simulink model "ss_ulin"  (Simulink 2.20)
settings: Solver=ode45  StartTime=0.0  StopTime=10.0  RelTol=1e-3  AbsTol=1e-6
values from neighbouring files (symbols this model uses):
  K = acker(Phi, Gamma, pz)    [tilstandmodel_lang_pind.m]
  k1 = 14.69268    [tilstandmodel_lang_pind.m]
  k2 = 1.43688    [tilstandmodel_lang_pind.m]
  k3 = 6.41894    [tilstandmodel_lang_pind.m]
  Keff = 1.3146    [tilstandmodel_lang_pind.m]
  kr1 = Phi_r(2,1)-Lr*Phi_r(1,1)    [tilstandmodel_lang_pind.m]
  kr2 = Phi_r(2,2)-Lr*Phi_r(1,2)    [tilstandmodel_lang_pind.m]
  kr3 = Gamma_r(2)-Lr*Gamma_r(1)    [tilstandmodel_lang_pind.m]
  Lr = (Phi_r(2,2) -pze)/Phi_r(1,2)    [tilstandmodel_lang_pind.m]
  N1 = 14/40    (= 0.35)    [tilstandmodel_lang_pind.m]
  N2 = 12/40    (= 0.3)    [tilstandmodel_lang_pind.m]
libraries: simulink x2
settings Model: ConsistencyChecking=off  RTWPlaceOutputsASAP=off

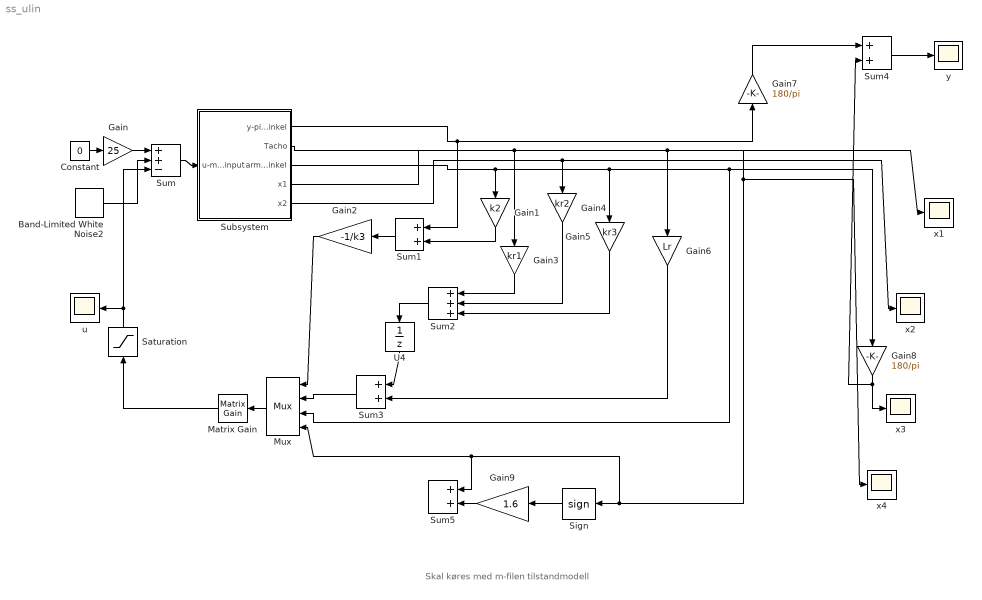
== system ss_ulin ==
  note: Skal køres med m-filen tilstandmodell
  Band-Limited White Noise2 : simulink/Sources/Band-Limited White Noise  Cov=[0.2]  Ts=0.025  seed=[23341]
  Constant : Constant  Value=0
  Gain : Gain  Gain=25
  Gain1 : Gain  Orientation=down  Gain=k2
  Gain2 : Gain  Orientation=left  Gain=-1/k3
  Gain3 : Gain  Orientation=down  Gain=kr1
  Gain4 : Gain  Orientation=down  Gain=kr2
  Gain5 : Gain  Orientation=down  Gain=kr3
  Gain6 : Gain  Orientation=down  Gain=Lr
  Gain7 : Gain  Orientation=up  Gain=180/pi
  Gain8 : Gain  Orientation=down  Gain=180/pi
  Gain9 : Gain  Orientation=left  Gain=1.6
  Matrix Gain : simulink/Linear/Matrix Gain  Orientation=left  K=K
  Mux : Mux  Orientation=left  Inputs=4
  Saturation : Saturate  Orientation=up  UpperLimit=5  LowerLimit=-5
  Sign : Signum  Orientation=left
  Subsystem : Subsystem
  Sum : Sum  Inputs=++-
  Sum1 : Sum  Orientation=left  Inputs=++
  Sum2 : Sum  Orientation=left  Inputs=+++
  Sum3 : Sum  Orientation=left  Inputs=++
  Sum4 : Sum  Inputs=++
  Sum5 : Sum  Orientation=left  Inputs=++
  U4 : UnitDelay  Orientation=down  X0=0  SampleTime=0.025
  u : Scope
      settings: TickLabels=on  TimeRange=auto  YMin=-5  YMax=5  SaveToWorkspace=off  SaveName=ScopeData  LimitMaxRows=off
  x{1..4} (4 alike) : Scope
      settings: TickLabels=on  TimeRange=auto  YMin=-5  YMax=5  SaveToWorkspace=off  SaveName=ScopeData  LimitMaxRows=off
  y : Scope
      settings: TickLabels=on  TimeRange=auto  YMin=-5  YMax=5  SaveToWorkspace=off  SaveName=ScopeData  LimitMaxRows=off
  wires:
  Constant/1 -> Gain/1
  Gain/1 -> Sum/1
  Gain1/1 -> Sum1/2
  Sum1/1 -> Gain2/1
  Mux/1 -> Matrix Gain/1
  Gain2/1 -> Mux/1
  Sum3/1 -> Mux/2
  Gain6/1 -> Sum3/2
  Sum2/1 -> U4/1
  U4/1 -> Sum3/1
  Gain3/1 -> Sum2/1
  Gain4/1 -> Sum2/2
  Gain5/1 -> Sum2/3
  Matrix Gain/1 -> Saturation/1
  Band-Limited White Noise2/1 -> Sum/2
  Gain7/1 -> Sum4/1
  Gain8/1 -> x3/1, Sum4/2
  Sum4/1 -> y/1
  Sum/1 -> Subsystem/1(u-motorinput)
  Saturation/1 -> Sum/3, u/1
  Subsystem/1(y-pindvinkel) -> Sum1/1, Gain7/1
  Subsystem/2(Tacho) -> x4/1, Sign/1, Sum5/1, Mux/4
  Subsystem/3(arm vinkel) -> Gain1/1, Mux/3, Gain8/1, Gain5/1
  Subsystem/4(x1) -> Gain3/1, x1/1, Gain6/1
  Subsystem/5(x2) -> Gain4/1, x2/1
  Sign/1 -> Gain9/1
  Gain9/1 -> Sum5/2

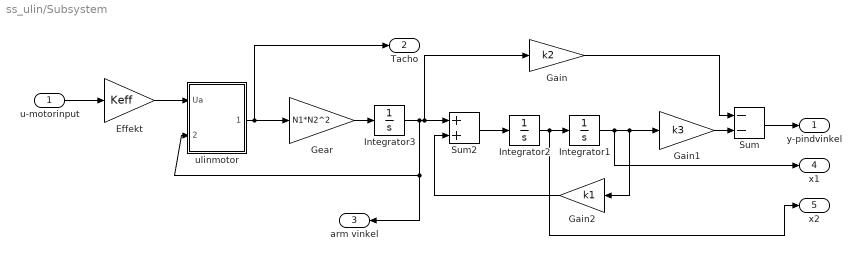
== system ss_ulin/Subsystem ==
  u-motorinput : Inport  Port=1  PortWidth=-1  SampleTime=-1
  Effekt : Gain  Gain=Keff
  Gain : Gain  Gain=k2
  Gain1 : Gain  Gain=k3
  Gain2 : Gain  Orientation=left  Gain=k1
  Gear : Gain  Gain=N1*N2^2
  Integrator1 : Integrator  ExternalReset=none  InitialConditionSource=internal  InitialCondition=0  LimitOutput=off  UpperSaturationLimit=inf  LowerSaturationLimit=-inf  ShowSaturationPort=off  ShowStatePort=off  AbsoluteTolerance=auto
  Integrator2 : Integrator  ExternalReset=none  InitialConditionSource=internal  InitialCondition=0  LimitOutput=off  UpperSaturationLimit=inf  LowerSaturationLimit=-inf  ShowSaturationPort=off  ShowStatePort=off  AbsoluteTolerance=auto
  Integrator3 : Integrator  ExternalReset=none  InitialConditionSource=internal  InitialCondition=0  LimitOutput=off  UpperSaturationLimit=inf  LowerSaturationLimit=-inf  ShowSaturationPort=off  ShowStatePort=off  AbsoluteTolerance=auto
  Sum : Sum  Inputs=--
  Sum2 : Sum  Inputs=++
  ulinmotor : Subsystem
  y-pindvinkel : Outport  Port=1  InitialOutput=0
  Tacho : Outport  Port=2  InitialOutput=0
  arm vinkel : Outport  Orientation=left  Port=3  InitialOutput=0
  x1 : Outport  Port=4  InitialOutput=0
  x2 : Outport  Port=5  InitialOutput=0
  wires:
  u-motorinput/1 -> Effekt/1
  Sum2/1 -> Integrator2/1
  Gain2/1 -> Sum2/2
  Gain1/1 -> Sum/2
  Gain/1 -> Sum/1
  Sum/1 -> y-pindvinkel/1
  Gear/1 -> Integrator3/1
  Integrator3/1 -> Sum2/1, Gain/1, arm vinkel/1, ulinmotor/2(Theta_a)
  Effekt/1 -> ulinmotor/1(Ua)
  ulinmotor/1(Omega) -> Gear/1, Tacho/1
  Integrator1/1 -> Gain1/1, Gain2/1, x1/1
  Integrator2/1 -> Integrator1/1, x2/1

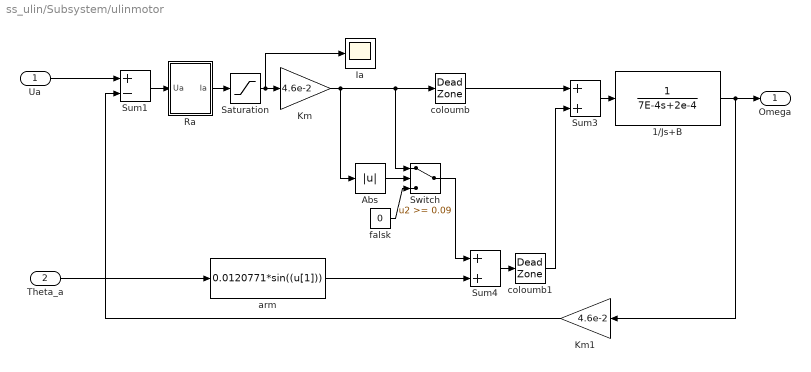
== system ss_ulin/Subsystem/ulinmotor ==
  Ua : Inport  Port=1  PortWidth=-1  SampleTime=-1
  Theta_a : Inport  Port=2  PortWidth=-1  SampleTime=-1
  1/Js+B : TransferFcn  Numerator=[1]  Denominator=[7E-4 2e-4]
  Abs : Abs
  Ia : Scope
      settings: TickLabels=on  TimeRange=5  YMin=-3  YMax=3  SaveToWorkspace=off  SaveName=ScopeData
  Km : Gain  Gain=4.6e-2
  Km1 : Gain  Orientation=left  Gain=4.6e-2
  Ra : Subsystem
  Saturation : Saturate  UpperLimit=6.5  LowerLimit=-6.5
  Sum1 : Sum  Inputs=+-
  Sum3 : Sum  Inputs=++
  Sum4 : Sum  Inputs=++
  Switch : Switch  Threshold=0.09
  arm : Fcn  Expr=0.0120771*sin((u[1]))
  coloumb : DeadZone  LowerValue=-0.09  UpperValue=0.09
  coloumb1 : DeadZone  LowerValue=-2.857  UpperValue=2.857
  falsk : Constant  Value=0
  Omega : Outport  Port=1  InitialOutput=0
  wires:
  Sum3/1 -> 1/Js+B/1
  Ua/1 -> Sum1/1
  Sum1/1 -> Ra/1(Ua)
  Theta_a/1 -> arm/1
  1/Js+B/1 -> Omega/1, Km1/1
  coloumb/1 -> Sum3/1
  coloumb1/1 -> Sum3/2
  arm/1 -> Sum4/2
  Sum4/1 -> coloumb1/1
  Km/1 -> Abs/1, coloumb/1, Switch/1
  Abs/1 -> Switch/2
  falsk/1 -> Switch/3
  Switch/1 -> Sum4/1
  Ra/1(Ia) -> Saturation/1
  Saturation/1 -> Km/1, Ia/1
  Km1/1 -> Sum1/2

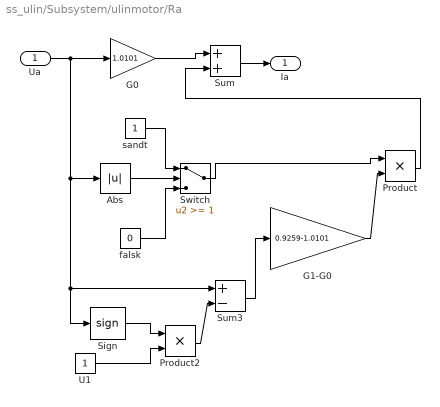
== system ss_ulin/Subsystem/ulinmotor/Ra ==
  Ua : Inport  Port=1  PortWidth=-1  SampleTime=-1
  Abs : Abs
  G0 : Gain  Gain=1.0101
  G1-G0 : Gain  Gain=0.9259-1.0101
  Product : Product  Inputs=2
  Product2 : Product  Inputs=2
  Sign : Signum
  Sum : Sum  Inputs=++
  Sum3 : Sum  Inputs=+-
  Switch : Switch  Threshold=1
  U1 : Constant  Value=1
  falsk : Constant  Value=0
  sandt : Constant  Value=1
  Ia : Outport  Port=1  InitialOutput=0
  wires:
  Product/1 -> Sum/2
  G1-G0/1 -> Product/2
  Sum3/1 -> G1-G0/1
  Product2/1 -> Sum3/2
  U1/1 -> Product2/2
  Sign/1 -> Product2/1
  Switch/1 -> Product/1
  sandt/1 -> Switch/1
  falsk/1 -> Switch/3
  Abs/1 -> Switch/2
  Ua/1 -> Sign/1, Sum3/1, Abs/1, G0/1
  G0/1 -> Sum/1
  Sum/1 -> Ia/1
